simulink model "model2"  (Simulink 7.9)
settings: Solver=ode45  StartTime=0.0  StopTime=Tsim  RelTol=1e-3
values from neighbouring files (symbols this model uses):
  Asin = 1    [script.m]    (also in script1.m; script2.m; script2Q3.m)
  Fsin1 = 2*pi*(85*10^3)    (= 534070.75111)    [script2.m]    (also in script2Q3.m = 534107.821904)
  Fsin2 = 2*pi*(90*10^3)    (= 565486.677646)    [script2.m]    (also in script2Q3.m)
  Fsin3 = 2*pi*(95*10^3)    (= 596902.604182)    [script2.m]    (also in script2Q3.m = 596819.666136)
  Fsin4 = 2*pi*(100*10^3)    (= 628318.530718)    [script2.m]    (also in script2Q3.m)
  Fsin5 = 2*pi*(115*10^3)    (= 722566.310326)    [script2.m]    (also in script2Q3.m = 722666.212972)
  Fsin6 = 2*pi*(120*10^3)    (= 753982.236862)    [script2.m]    (also in script2Q3.m = 0)
  Te = T/M    (= 0.03125)    [script.m]    (also in script1.m; script2.m = 3.125e-06; script2Q3.m = 3.125e-06)
settings Model: Creator=pamaury  LastModifiedBy=pamaury

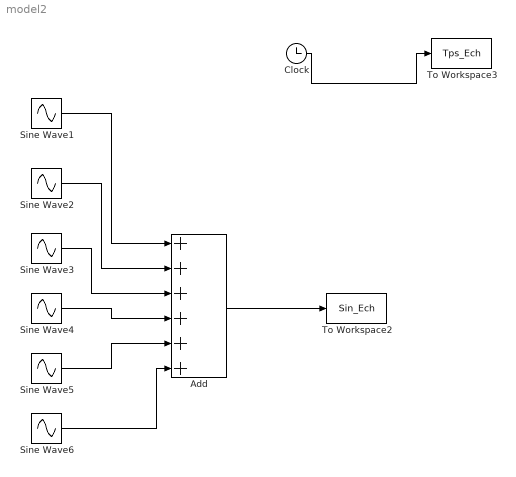
== system model2 ==
  Add : Sum  Inputs=++++++
  Clock : Clock
  Sine Wave1 : Sin  Amplitude=Asin  Frequency=Fsin1  SampleTime=0
  Sine Wave2 : Sin  Amplitude=Asin  Frequency=Fsin2  SampleTime=0
  Sine Wave3 : Sin  Amplitude=Asin  Frequency=Fsin3  SampleTime=0
  Sine Wave4 : Sin  Amplitude=Asin  Frequency=Fsin4  SampleTime=0
  Sine Wave5 : Sin  Amplitude=Asin  Frequency=Fsin5  SampleTime=0
  Sine Wave6 : Sin  Amplitude=Asin  Frequency=Fsin6  SampleTime=0
  To Workspace2 : ToWorkspace  VariableName=Sin_Ech  SampleTime=Te
  To Workspace3 : ToWorkspace  VariableName=Tps_Ech  SampleTime=Te
  wires:
  Clock/1 -> To Workspace3/1
  Add/1 -> To Workspace2/1
  Sine Wave1/1 -> Add/1
  Sine Wave2/1 -> Add/2
  Sine Wave3/1 -> Add/3
  Sine Wave4/1 -> Add/4
  Sine Wave5/1 -> Add/5
  Sine Wave6/1 -> Add/6
